simulink model "Kalman"  (R2025b)
settings: Solver=VariableStepAuto  StartTime=0.0  StopTime=10.0  RelTol=1e-3
undefined symbols (not defined in the file): C, ic_yz, K_vert, sysKF
settings Model: Creator=JPham  LastModifiedBy=JPham

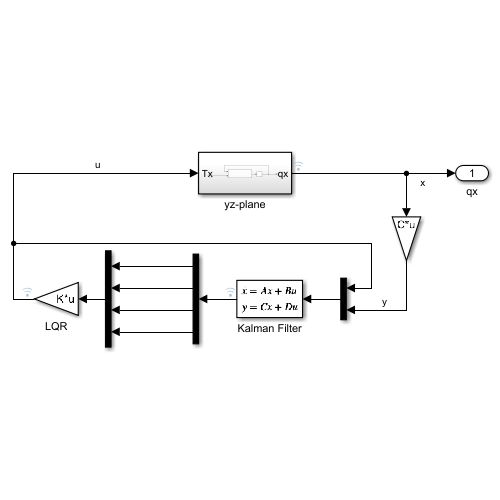
[thumbnail: Simulink's stored preview of the top-level diagram]
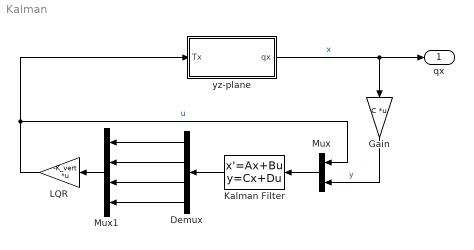
== system Kalman ==
  Demux : Demux
  Gain : Gain  Gain=C  Multiplication=Matrix(K*u)
  Kalman Filter : StateSpace  A=sysKF.A  B=sysKF.B  C=sysKF.C  D=sysKF.D  InitialCondition=ic_yz
  LQR : Gain  Gain=-K_vert  Multiplication=Matrix(K*u)
  Mux : Mux  Inputs=2
  Mux1 : Mux
  yz-plane : Subsystem
  qx : Outport
  wires:
  yz-plane/1(qx) -> qx/1, Gain/1  "x"
  LQR/1 -> yz-plane/1(Tx), Mux/1  "u"
  Gain/1 -> Mux/2  "y"
  Mux/1 -> Kalman Filter/1
  Kalman Filter/1 -> Demux/1
  Mux1/1 -> LQR/1
  Demux/1 -> Mux1/1
  Demux/2 -> Mux1/2
  Demux/3 -> Mux1/3
  Demux/4 -> Mux1/4

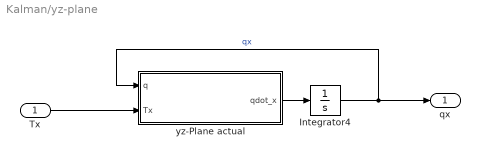
== system Kalman/yz-plane ==
  Tx : Inport
  Integrator4 : Integrator  InitialCondition=ic_yz  ContinuousStateAttributes='angle'
  yz-Plane actual : MATLAB Function  TreatAsAtomicUnit=on
  qx : Outport
  wires:
  Tx/1 -> yz-Plane actual/2(Tx)
  yz-Plane actual/1(qdot_x) -> Integrator4/1
  Integrator4/1 -> qx/1, yz-Plane actual/1(q)  "qx"

== matlab function Kalman/yz-plane/yz-Plane actual ==
  data: q input; Tx input; qdot_x output
function qdot_x = f(q, Tx)
    % Define dimensions for code generation
    % x is 4x1 state: [phi; theta; phi_dot; theta_dot]
    % Tm is the torque from the three motors
    % p is the parameter structure, loaded into simulink in Model Explorer

    % Convert motor torque to omniwheel torque
    alpha = params().alpha;
    beta  = params().beta;
    % Tx = cos(alpha)*(Tm(1)*cos(beta)) - Tm(2)*sin(beta + pi/6) + Tm(3)*sin(beta - pi/6);

    % States
    phi     = q(1); % phi
    theta   = q(2); % theta
    dotphi  = q(3); % phi_dot
    dottheta= q(4); % theta_dot
    
    p = params;
    % Aux Parameters
    m_tot = p.m_ball + p.m_body + p.m_virt;
    r_tot = p.r_ball + p.r_omni;
    gamma = p.l*p.m_body + (p.r_ball + p.r_omni)*p.m_virt;
    
    % M matrix
    M11 = m_tot * p.r_ball^2 + p.Theta_ball + (p.r_ball / p.r_omni)^2 * p.Theta_virt_vertical;
    M12 = -(p.r_ball / p.r_omni^2) * r_tot * p.Theta_virt_vertical + gamma * p.r_ball*cos(theta); 
    M22 = (r_tot^2 / p.r_omni^2) * p.Theta_virt_vertical + p.Theta_body_vertical + ...
           p.m_body * p.l^2 + p.m_virt * r_tot^2;
    M21 = M12;

    M = [M11, M12;
         M21, M22];
    
    % C vector
    Cvec = [ -p.r_ball*gamma*sin(theta)*dottheta^2; 
              0 ];
    % G vector
    Gvec = [ 0; 
            -p.g*sin(theta)*gamma ];
    % S vector (f_NP = S*u(t))
    S = [ p.r_ball / p.r_omni; -p.r_ball / p.r_omni ];
    
    % --- Dynamics Calculation ---
    F_np = S * Tx; 
    
    % Solve for qdd from M * qdd + C + G = F_np
    % qddot = M \ (F_np - C - G) = [theta_doubledot; phi_doubledot]
    qddot = M \ (F_np - Cvec - Gvec);
    
    % Assemble qdot_vertical
    qdot_x = [dotphi;
              dottheta;
              qddot(1);
              qddot(2)];
end
